simulink model "cruise_control_sys"  (R2016b)
settings: Solver=VariableStepAuto  StartTime=0.0  StopTime=100  RelTol=1e-3
values from neighbouring files (symbols this model uses):
  A = -b/m    (= -0.05)    [work.m]
  B = 1/m    (= 0.001)    [work.m]
  C = 1    [work.m]
  D = 0    [work.m]
  Kd = 20    [work.m]
  Ki = 15    [work.m]
  Kp = 300    [work.m]
settings Model: Creator=BlakelyMayhall  LastModifiedBy=BlakelyMayhall

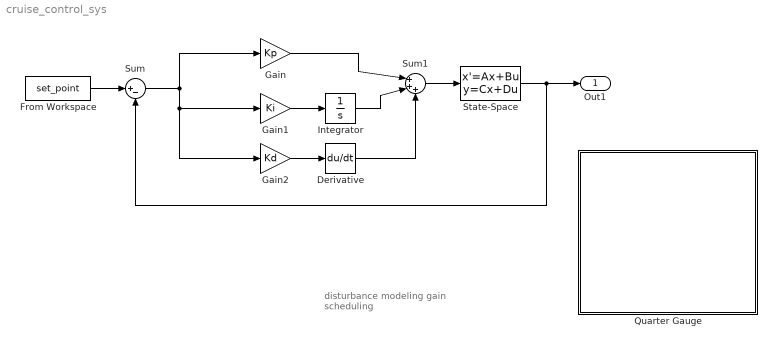
== system cruise_control_sys ==
  note: disturbance modeling
      | gain scheduling
  Derivative : Derivative
  From Workspace : FromWorkspace  VariableName=set_point  SampleTime=0
  Gain : Gain  Gain=Kp
  Gain1 : Gain  Gain=Ki
  Gain2 : Gain  Gain=Kd
  Integrator : Integrator
  Quarter Gauge : Subsystem  DialogController=hmiCreateDDGDialog  IsWebBlock=on  mask(MWDashboardBlock){webBlockId=df28eaef-f424-479e-8e68-14f6f797f306, webBlockType=ninetydegreegauge, ShowInLibBrowser=on, ShowInitialText=on, HMISrcModelName=cruise_control_sys}
      mask prompts: webBlockId "WebBlock Id"; webBlockType "WebBlock Type"; HMISrcModelName "Source Model"
      mask help: SimulinkHMI:dialogs:NinetydegreeGaugeDialogDesc
      mask Help: helpview([docroot '/mapfiles/simulink.map'], 'hmi_quarter_gauge')
      mask Display:
      | if strcmp(get_param(bdroot(gcb),'BlockDiagramType'), 'library')
      |     image([(matlabroot) '/toolbox/simulink/hmi/icons/NinetyDegreeGauge.png']);
      | end
  State-Space : StateSpace  A=A  B=B  C=C  D=D  X0=50
  Sum : Sum  Inputs=|+-
  Sum1 : Sum  Inputs=|+++
  Out1 : Outport  SignalName=u
  wires:
  Sum/1 -> Gain2/1, Gain1/1, Gain/1
  From Workspace/1 -> Sum/1
  Gain2/1 -> Derivative/1
  Gain1/1 -> Integrator/1
  Gain/1 -> Sum1/1
  Integrator/1 -> Sum1/2
  Derivative/1 -> Sum1/3
  Sum1/1 -> State-Space/1
  State-Space/1 -> Out1/1, Sum/2

== system cruise_control_sys/Quarter Gauge ==
